simulink model "AS_H_Balanced_Load_7Bus"  (R2021a)
settings: Solver=ode45  StartTime=0.0  StopTime=1  RelTol=1e-3  EnableMultiTasking=on
undefined symbols (not defined in the file): D1, Delta
libraries: simulink_extras x12, spsDCVoltageSourceLib x12, spsDiodeLib x12, spsSeriesRLCBranchLib x12, spsGroundLib x10, spsRMSLib x8, dspstat3 x7, spsThreePhaseTransformerTwoWindingsLib x7, spsBreakerLib x7, spsThreePhaseSeriesRLCBranchLib x6, spsThreePhaseParallelRLCLoadLib x5, eePMU x4
(part 1 of 2)
settings Model: Creator=Gajanan-pc  LastModifiedBy=Hewlett-packard
settings SolverCC: AlgebraicLoopSolver=TrustRegion
settings DataIOCC: LimitDataPoints=on  SaveFormat=Array  ReturnWorkspaceOutputs=off
settings OptimizationCC: LifeSpan=inf
settings DebuggingCC: MaxConsecutiveZCsMsg=none  SolverPrmCheckMsg=warning  ParameterPrecisionLossMsg=none  SFUnexpectedBacktrackingDiag=warning  SFNoUnconditionalDefaultTransitionDiag=warning  SFExecutionAtInitializationDiag=none  SFMachineParentedDataDiag=warning  ArithmeticOperatorsInVariantConditions=warning
settings HardwareCC: ProdBitPerPointer=32  ProdBitPerSizeT=32  ProdBitPerPtrDiffT=32  ProdLargestAtomicFloat=None  ProdIntDivRoundTo=Undefined  ProdEndianess=Unspecified  ProdWordSize=32  ProdHWDeviceType=32-bit Generic
settings ModelReferenceCC: PropagateSignalLabelsOutOfModel=off
settings SFSimCC: SimUseLocalCustomCode=off  CustomCodeUndefinedFunction=UseInterfaceOnly
settings RTWCC: RTWUseLocalCustomCode=off
settings CodeAppCC: StateflowObjectComments=on
settings GRTTargetCC: TargetLangStandard=C89/C90 (ANSI)
settings ConfigComp: CovMetricSettings=dw  CovSaveCumulativeToWorkspaceVar=on  CovSaveSingleToWorkspaceVar=on  CovExternalEMLEnable=off  CovSFcnEnable=off
settings SimscapeCC: SimscapeNormalizeSystem=off

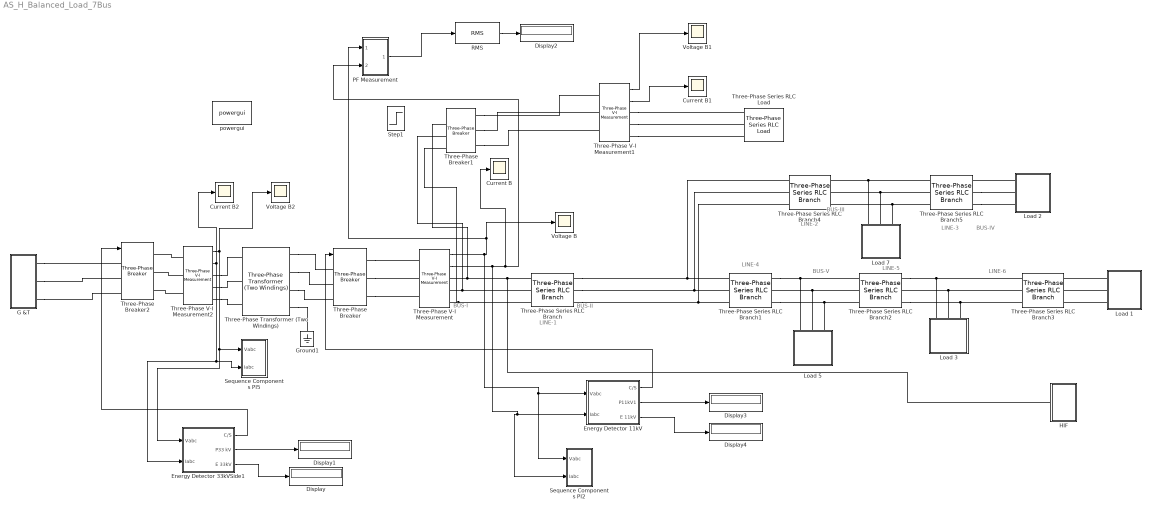
== system AS_H_Balanced_Load_7Bus ==
  note: LINE-1
  note: BUS-I
  note: BUS-II
  note: BUS-III
  note: BUS-IV
  note: BUS-V
  note: LINE-2
  note: LINE-3
  note: LINE-4
  note: LINE-5
  note: LINE-6
  Current B : Scope
  Current B1 : Scope
  Current B2 : Scope
  Display{,1..4} (5 alike) : Display
  Energy Detector 11kV : Subsystem
  Energy Detector 33kVSide1 : Subsystem
  G &T : Subsystem
  Ground1 : spsGroundLib/Ground  LConnTagsString=a
  HIF : Subsystem
  Load 1 : Subsystem
  Load 2 : Subsystem
  Load 3 : Subsystem
  Load 5 : Subsystem
  Load 7 : Subsystem
  PF Measurement : Subsystem
  RMS : dspstat3/RMS  run=off  directionMode=Each column  dimension=1  InputProcessing=Columns as channels (frame based)  reset_popup=None
  Sequence Components PI2 : Subsystem
  Sequence Components PI5 : Subsystem
  Step1 : Step  Time=0.8  SampleTime=0.1  ZeroCross=off
  Three-Phase Series RLC Branch : spsThreePhaseSeriesRLCBranchLib/Three-Phase Series RLC Branch  LConnTagsString=A|B|C  RConnTagsString=A|B|C  BranchType=RL  Resistance=0.2232  Inductance=0.012  Capacitance=0  Measurements=None
  Three-Phase Series RLC Branch1 : spsThreePhaseSeriesRLCBranchLib/Three-Phase Series RLC Branch  LConnTagsString=A|B|C  RConnTagsString=A|B|C  BranchType=RL  Resistance=0.9207  Inductance=0.0495  Capacitance=0  Measurements=None
  Three-Phase Series RLC Branch2 : spsThreePhaseSeriesRLCBranchLib/Three-Phase Series RLC Branch  LConnTagsString=A|B|C  RConnTagsString=A|B|C  BranchType=RL  Resistance=0.6138  Inductance=0.033  Capacitance=0  Measurements=None
  Three-Phase Series RLC Branch3 : spsThreePhaseSeriesRLCBranchLib/Three-Phase Series RLC Branch  LConnTagsString=A|B|C  RConnTagsString=A|B|C  BranchType=RL  Resistance=1.602  Inductance=0.057  Capacitance=0  Measurements=None
  Three-Phase Series RLC Branch4 : spsThreePhaseSeriesRLCBranchLib/Three-Phase Series RLC Branch  LConnTagsString=A|B|C  RConnTagsString=A|B|C  BranchType=RL  Resistance=0.7812  Inductance=0.042  Capacitance=0  Measurements=None
  Three-Phase Series RLC Branch5 : spsThreePhaseSeriesRLCBranchLib/Three-Phase Series RLC Branch  LConnTagsString=A|B|C  RConnTagsString=A|B|C  BranchType=RL  Resistance=1.1997  Inductance=0.0645  Capacitance=0  Measurements=None
  Three-Phase Series RLC Load : spsThreePhaseSeriesRLCLoadLib/Three-Phase Series RLC Load  LConnTagsString=A|B|C  Configuration=Y (floating)  NominalVoltage=12.65e3  Vabc=[1e3 1e3 1e3]  Vabcp=[1e3 1e3 1e3]  NominalFrequency=50  UnbalancedPower=off  ActivePower=0  InductivePower=108e3  CapacitivePower=1800e3  Pabc=[10e3 9e3 11e3]  QLabc=[100 90 110]  QCabc=[100 90 110]  Pabcp=[10e3 9e3 11e3]  QLabcp=[100 90 110]  QCabcp=[100 90 110]  Measurements=Branch voltages and currents  LoadType=constant PQ
  Three-Phase Transformer (Two Windings) : spsThreePhaseTransformerTwoWindingsLib/Three-Phase Transformer (Two Windings)  Winding1Connection=Delta (D1)  Winding2Connection=Yn  CoreType=Three-limb core (core-type)  SetSaturation=off  Hysteresis=off  DataFile='hysteresis'  SetInitialFlux=off  Measurements=None  UNITS=pu  NominalPower=[ 10e6 , 50 ]  Winding1=[33e3 , 0.002 , 0.08 ]  Winding2=[11e3 , 0.002 , 0.08 ]  Rm=500  Lm=500  L0=0.5  Saturation=[ 0,0 ; 0.0024,1.2 ; 1.0,1.52 ]  InitialFluxes=[-0.84855560977397 0.870082768362299 -0.0215271585931069]  BreakLoop=off  DiscreteSolver=Trapezoidal iterative  DataType=off  TransfoNumber=1
  Three-Phase V-I Measurement : spsThreePhaseVIMeasurementLib/Three-Phase V-I Measurement  VoltageMeasurement=phase-to-phase  SetLabelV=off  LabelV=Vabc  Vpu=off  VpuLL=off  CurrentMeasurement=yes  SetLabelI=off  LabelI=Iabc  Ipu=off  Pbase=100e6  Vbase=11e3  OutputType=Complex  PhasorSimulation=off  PSBequivalent=0
  Three-Phase V-I Measurement1 : spsThreePhaseVIMeasurementLib/Three-Phase V-I Measurement  VoltageMeasurement=phase-to-phase  SetLabelV=off  LabelV=Vabc  Vpu=off  VpuLL=off  CurrentMeasurement=yes  SetLabelI=off  LabelI=Iabc  Ipu=off  Pbase=100e6  Vbase=11e3  OutputType=Complex  PhasorSimulation=off  PSBequivalent=0
  Three-Phase V-I Measurement2 : spsThreePhaseVIMeasurementLib/Three-Phase V-I Measurement  VoltageMeasurement=phase-to-phase  SetLabelV=off  LabelV=Vabc  Vpu=off  VpuLL=off  CurrentMeasurement=yes  SetLabelI=off  LabelI=Iabc  Ipu=off  Pbase=100e6  Vbase=11e3  OutputType=Complex  PhasorSimulation=off  PSBequivalent=0
  Three-Phase Breaker : spsThreePhaseBreakerLib/Three-Phase Breaker  InitialState=closed  SwitchA=on  SwitchB=on  SwitchC=on  SwitchTimes=[1/50 5/50]  External=on  BreakerResistance=0.01  SnubberResistance=1e6  SnubberCapacitance=inf  Measurements=Breaker voltages and currents
  Three-Phase Breaker1 : spsThreePhaseBreakerLib/Three-Phase Breaker  InitialState=closed  SwitchA=on  SwitchB=on  SwitchC=on  SwitchTimes=[1/50 5/50]  External=on  BreakerResistance=0.01  SnubberResistance=1e6  SnubberCapacitance=inf  Measurements=Breaker voltages and currents
  Three-Phase Breaker2 : spsThreePhaseBreakerLib/Three-Phase Breaker  InitialState=closed  SwitchA=on  SwitchB=on  SwitchC=on  SwitchTimes=[1/50 5/50]  External=on  BreakerResistance=0.01  SnubberResistance=1e6  SnubberCapacitance=inf  Measurements=Breaker voltages and currents
  Voltage B : Scope
  Voltage B1 : Scope
  Voltage B2 : Scope
  powergui : spspowerguiLib/powergui  Priority=1  SimulationMode=Discrete  SampleTime=50e-6  frequency=60  Iterations=50  frequencyindice=0  Pbase=100e6  ErrMax=0.0001  UnitsV=kV  UnitsW=MW  buscounter=0  FunctionMessages=off  echomessages=off  EnableUseOfTLC=off  CurrentSourceSwitches=off  DisableSnubberDevices=off  DisableRonSwitches=off  DisableVfSwitches=off  DisplayEquations=off  AutomaticDiscreteSolvers=off  SolverType=Backward Euler  Interpol=off  ExternalGateDelay=off  methode=off  Ts=0  x0status=blocks  SPID=off  SwTol=0  HookPort=off  NonlinearTolerance=0  nMaxIteration=15  ContinueOnMaxIteration=off  RestoreLinks=warning  ResistiveCurrentMeasurement=off  Frange=[0:2:500]  Ylog=off  Xlog=on  ShowGrid=off  save=off  variable=ZData  structure=0  ZoomFFT=off  StartTime=0.0  cycles=1  DisplayStyle=1  fundamental=60  FreqAxis=off  MaxFrequency=1000  frequencyindicesteady=1  RmsSteady=1  display=off
  wires:
  Three-Phase V-I Measurement/2 -> Sequence Components PI2/2(Iabc), Energy Detector 11kV/2(Iabc), Current B/1, PF Measurement/2(In2)
  Three-Phase V-I Measurement1/1 -> Voltage B1/1
  Three-Phase V-I Measurement1/2 -> Current B1/1
  RMS/1 -> Display2/1
  PF Measurement/1(Out1) -> RMS/1
  Energy Detector 11kV/1(C/S) -> Three-Phase Breaker/1
  Three-Phase V-I Measurement/1 -> Sequence Components PI2/1(Vabc), Energy Detector 11kV/1(Vabc), Voltage B/1, PF Measurement/1(In1)
  Three-Phase V-I Measurement2/1 -> Sequence Components PI5/1(Vabc), Energy Detector 33kVSide1/1(Vabc), Voltage B2/1
  Three-Phase V-I Measurement2/2 -> Energy Detector 33kVSide1/2(Iabc), Sequence Components PI5/2(Iabc), Current B2/1
  Energy Detector 33kVSide1/1(C/S) -> Three-Phase Breaker2/1
  Energy Detector 33kVSide1/3(E 33kV) -> Display/1
  Energy Detector 33kVSide1/2(P33 kV) -> Display1/1
  Energy Detector 11kV/2(P11kV1) -> Display3/1
  Energy Detector 11kV/3(E 11kV) -> Display4/1
  connections:
  Three-Phase Series RLC Branch3/LConn2 -- Three-Phase Series RLC Branch2/RConn2 -- Load 3/LConn2
  Three-Phase Series RLC Branch2/RConn3 -- Load 3/LConn3 -- Three-Phase Series RLC Branch3/LConn3
  Three-Phase Series RLC Branch/LConn2 -- Three-Phase Breaker1/LConn2 -- Three-Phase V-I Measurement/RConn2
  Three-Phase Breaker/RConn2 -- Three-Phase V-I Measurement/LConn2
  Three-Phase Series RLC Branch/RConn3 -- Three-Phase Series RLC Branch1/LConn3 -- Three-Phase Series RLC Branch4/LConn3
  Three-Phase Series RLC Branch/LConn3 -- Three-Phase Breaker1/LConn3 -- Three-Phase V-I Measurement/RConn3
  Three-Phase Breaker/RConn1 -- Three-Phase V-I Measurement/LConn1
  Three-Phase Breaker/RConn3 -- Three-Phase V-I Measurement/LConn3
  Three-Phase Series RLC Branch5/LConn2 -- Load 7/LConn2 -- Three-Phase Series RLC Branch4/RConn2
  Three-Phase Series RLC Branch5/LConn3 -- Load 7/LConn3 -- Three-Phase Series RLC Branch4/RConn3
  Three-Phase Series RLC Branch/LConn1 -- HIF/LConn1 -- Three-Phase Breaker1/LConn1 -- Three-Phase V-I Measurement/RConn1
  Three-Phase Series RLC Branch1/RConn3 -- Three-Phase Series RLC Branch2/LConn3 -- Load 5/LConn3
  Three-Phase Series RLC Branch/RConn1 -- Three-Phase Series RLC Branch1/LConn1 -- Three-Phase Series RLC Branch4/LConn1
  Three-Phase V-I Measurement1/RConn1 -- Three-Phase Series RLC Load/LConn1
  Three-Phase V-I Measurement1/RConn2 -- Three-Phase Series RLC Load/LConn2
  Three-Phase V-I Measurement1/RConn3 -- Three-Phase Series RLC Load/LConn3
  Three-Phase Breaker1/RConn1 -- Three-Phase V-I Measurement1/LConn1
  Three-Phase Breaker1/RConn2 -- Three-Phase V-I Measurement1/LConn2
  Three-Phase Breaker1/RConn3 -- Three-Phase V-I Measurement1/LConn3
  Three-Phase Series RLC Branch2/LConn2 -- Load 5/LConn2 -- Three-Phase Series RLC Branch1/RConn2
  Three-Phase Series RLC Branch1/LConn2 -- Three-Phase Series RLC Branch4/LConn2 -- Three-Phase Series RLC Branch/RConn2
  Three-Phase Transformer (Two Windings)/RConn2 -- Three-Phase Breaker/LConn2
  Three-Phase Transformer (Two Windings)/RConn1 -- Three-Phase Breaker/LConn1
  Three-Phase Transformer (Two Windings)/RConn3 -- Three-Phase Breaker/LConn3
  Three-Phase Series RLC Branch5/LConn1 -- Three-Phase Series RLC Branch4/RConn1 -- Load 7/LConn1
  Load 1/LConn2 -- Three-Phase Series RLC Branch3/RConn2
  Load 1/LConn3 -- Three-Phase Series RLC Branch3/RConn3
  Load 2/LConn1 -- Three-Phase Series RLC Branch5/RConn1
  Three-Phase Series RLC Branch5/RConn2 -- Load 2/LConn2
  Three-Phase Series RLC Branch5/RConn3 -- Load 2/LConn3
  Three-Phase Transformer (Two Windings)/RConn4 -- Ground1/LConn1
  Load 1/LConn1 -- Three-Phase Series RLC Branch3/RConn1
  Load 5/LConn1 -- Three-Phase Series RLC Branch1/RConn1 -- Three-Phase Series RLC Branch2/LConn1
  Three-Phase V-I Measurement2/LConn1 -- Three-Phase Breaker2/RConn1
  Three-Phase V-I Measurement2/LConn2 -- Three-Phase Breaker2/RConn2
  Three-Phase V-I Measurement2/LConn3 -- Three-Phase Breaker2/RConn3
  Three-Phase V-I Measurement2/RConn1 -- Three-Phase Transformer (Two Windings)/LConn1
  Three-Phase V-I Measurement2/RConn2 -- Three-Phase Transformer (Two Windings)/LConn2
  Three-Phase V-I Measurement2/RConn3 -- Three-Phase Transformer (Two Windings)/LConn3
  G &T/RConn1 -- Three-Phase Breaker2/LConn1
  G &T/RConn2 -- Three-Phase Breaker2/LConn2
  G &T/RConn3 -- Three-Phase Breaker2/LConn3
  Three-Phase Series RLC Branch2/RConn1 -- Load 3/LConn1 -- Three-Phase Series RLC Branch3/LConn1

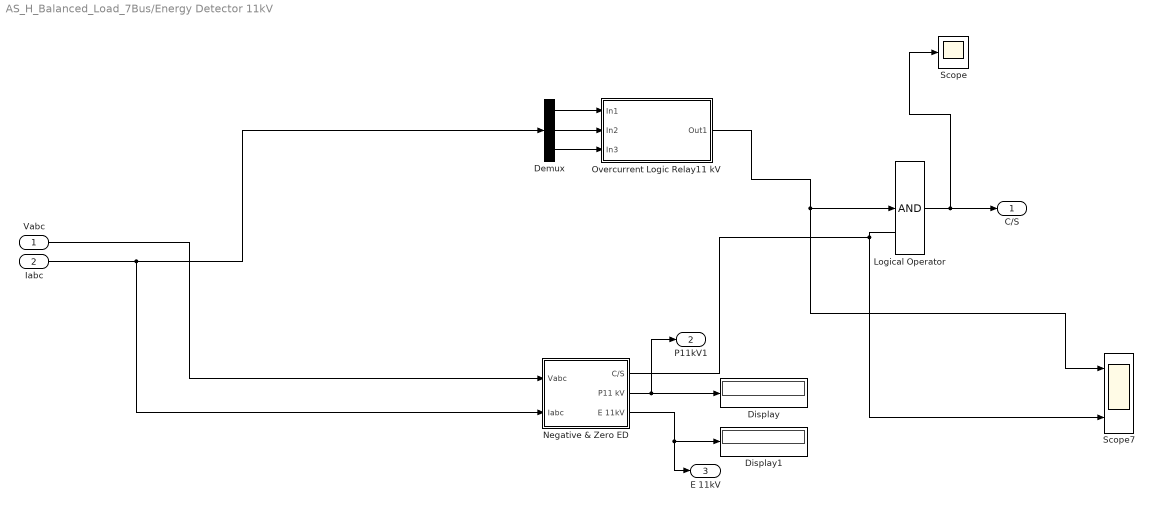
== system AS_H_Balanced_Load_7Bus/Energy Detector 11kV ==
  Vabc : Inport
  Iabc : Inport  Port=2
  Demux : Demux  Outputs=3
  Display : Display
  Display1 : Display
  Logical Operator : Logic  Inputs=1  AllPortsSameDT=off
  "Negative & Zero ED " : Subsystem
  "Overcurrent Logic Relay11 kV " : Subsystem  TreatAsAtomicUnit=on
  Scope : Scope
  Scope7 : Scope  NumInputPorts=3
  C/S : Outport  VectorParamsAs1DForOutWhenUnconnected=off
  P11kV1 : Outport  Port=2  VectorParamsAs1DForOutWhenUnconnected=off
  E 11kV : Outport  Port=3  VectorParamsAs1DForOutWhenUnconnected=off
  wires:
  Iabc/1 -> "Negative & Zero ED "/2(Iabc), Demux/1
  Demux/3 -> "Overcurrent Logic Relay11 kV "/3(In3)
  Demux/1 -> "Overcurrent Logic Relay11 kV "/1(In1)
  Demux/2 -> "Overcurrent Logic Relay11 kV "/2(In2)
  "Overcurrent Logic Relay11 kV "/1(Out1) -> Scope7/1, Logical Operator/1
  Logical Operator/1 -> Scope/1, C/S/1
  Vabc/1 -> "Negative & Zero ED "/1(Vabc)
  "Negative & Zero ED "/1(C/S) -> Scope7/3
  "Negative & Zero ED "/2(P11 kV) -> Display/1, P11kV1/1
  "Negative & Zero ED "/3(E 11kV) -> E 11kV/1, Display1/1

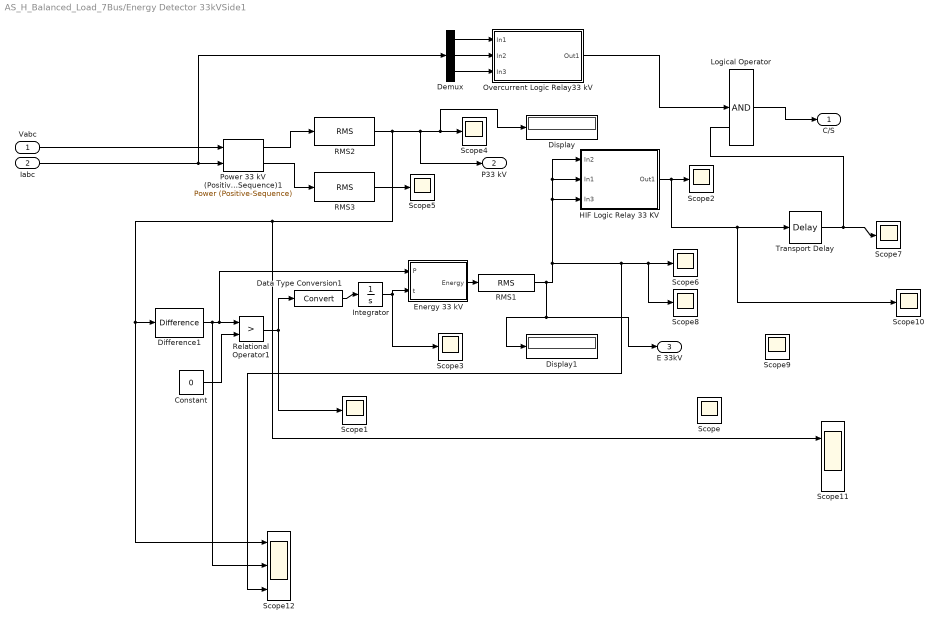
== system AS_H_Balanced_Load_7Bus/Energy Detector 33kVSide1 ==
  Vabc : Inport
  Iabc : Inport  Port=2
  Constant : Constant  Value=0
  Data Type Conversion1 : DataTypeConversion
  Demux : Demux  Outputs=3
  Difference1 : simulink/Discrete/Difference  ICPrevInput=0.0  OutMin=[]  OutMax=[]  OutDataType=fixdt(1, 16)  OutScaling=2^-10  DoSatur=off
  Display : Display
  Display1 : Display
  Energy 33 kV : MATLAB Function  TreatAsAtomicUnit=on
  HIF Logic Relay 33 KV : Subsystem  TreatAsAtomicUnit=on
  Integrator : Integrator
  Logical Operator : Logic  Inputs=1  AllPortsSameDT=off
  Overcurrent Logic Relay33 kV : Subsystem  TreatAsAtomicUnit=on
  Power 33 kV (Positive-Sequence)1 : spsPowerPositiveSequenceLib/Power (Positive-Sequence)  Freq=50  Vinit=[0, 0]  Iinit=[0, 0]  Ts=0
      link override Sequence Analyzer: Freq=50  seq=Negative
      link override Sequence Analyzer1: Freq=50  seq=Negative
      settings: SourceProductBaseCode=PS
  RMS1 : dspstat3/RMS  run=off  directionMode=Each column  dimension=1  InputProcessing=Columns as channels (frame based)  reset_popup=None
  RMS2 : dspstat3/RMS  run=off  directionMode=Each column  dimension=1  InputProcessing=Columns as channels (frame based)  reset_popup=None
  RMS3 : dspstat3/RMS  run=off  directionMode=Each column  dimension=1  InputProcessing=Columns as channels (frame based)  reset_popup=None
  Relational Operator1 : RelationalOperator  Operator=>  RndMeth=Nearest
  Scope{,1..10} (11 alike) : Scope
  Scope11 : Scope  NumInputPorts=2
  Scope12 : Scope  NumInputPorts=3
  Transport Delay : TransportDelay  DelayTime=0.1  InitialOutput=1
  C/S : Outport  VectorParamsAs1DForOutWhenUnconnected=off
  P33 kV : Outport  Port=2  VectorParamsAs1DForOutWhenUnconnected=off
  E 33kV : Outport  Port=3  VectorParamsAs1DForOutWhenUnconnected=off
  wires:
  Power 33 kV (Positive-Sequence)1/2 -> RMS3/1
  Iabc/1 -> Demux/1, Power 33 kV (Positive-Sequence)1/2
  Demux/3 -> Overcurrent Logic Relay33 kV/3(In3)
  RMS3/1 -> Scope5/1
  Demux/1 -> Overcurrent Logic Relay33 kV/1(In1)
  Energy 33 kV/1(Energy) -> RMS1/1
  Integrator/1 -> Scope3/1, Energy 33 kV/2(t)
  Power 33 kV (Positive-Sequence)1/1 -> RMS2/1
  Demux/2 -> Overcurrent Logic Relay33 kV/2(In2)
  Overcurrent Logic Relay33 kV/1(Out1) -> Logical Operator/1
  Vabc/1 -> Power 33 kV (Positive-Sequence)1/1
  Logical Operator/1 -> C/S/1
  Data Type Conversion1/1 -> Integrator/1
  Relational Operator1/1 -> Data Type Conversion1/1, Scope1/1
  RMS2/1 -> Scope11/1, Scope12/1, Difference1/1, P33 kV/1, Scope4/1, Display/1
  HIF Logic Relay 33 KV/1(Out1) -> Scope10/1, Transport Delay/1, Scope2/1
  Transport Delay/1 -> Scope7/1
  Constant/1 -> Relational Operator1/2
  Difference1/1 -> Scope12/2, Energy 33 kV/1(P), Relational Operator1/1
  RMS1/1 -> Display1/1, E 33kV/1, Scope12/3, Scope8/1, Scope6/1, HIF Logic Relay 33 KV/3(In3), HIF Logic Relay 33 KV/2(In1), HIF Logic Relay 33 KV/1(In2)

== system AS_H_Balanced_Load_7Bus/G &T ==
  Ground2 : spsGroundLib/Ground  LConnTagsString=a
  Ground3 : spsGroundLib/Ground  LConnTagsString=a
  Ground4 : spsGroundLib/Ground  LConnTagsString=a
  Three-Phase Programmable Voltage Source1 : spsThreePhaseProgrammableVoltageSourceLib/Three-Phase Programmable Voltage Source  PositiveSequence="[220e3  0 50]"  VariationEntity=None  VariationType=Table of time-amplitude pairs  VariationTypeAlt=Step  VariationStep=0.5  VariationRate=10  VariationMagnitude=0.3  VariationFrequency=2  VariationTiming=[.01 .05 1]  VariationPhaseA=off  Amplitudes=[1 0.8 1.2 1.0]  TimeValues=[0 0.1 0.15 0.2]  HarmonicGeneration=off  HarmonicA=[3 0.2 -25 0]  HarmonicB=[2 0.15 35 2]  Timing="[0.05  3]"  BusType=PQ  Pref=5e6  Qref=0  Qmin=0.5e6  Qmax=0
  Three-Phase Transformer (Two Windings)1 : spsThreePhaseTransformerTwoWindingsLib/Three-Phase Transformer (Two Windings)  Winding1Connection=Yn  Winding2Connection=Yn  CoreType=Three-limb core (core-type)  SetSaturation=off  Hysteresis=off  DataFile='hysteresis'  SetInitialFlux=off  Measurements=All measurements (V I Fluxes)  UNITS=pu  NominalPower=[ 50e6 , 50 ]  Winding1=[2.2e+05 0.002 0.08]  Winding2=[33000 0.002 0.08]  Rm=500  Lm=499.99  L0=0.49999  Saturation=[0 0;0.0024 1.2;1 1.52]  InitialFluxes=[-0.991141122701691 0.498581403361155 0.49255971934211]  BreakLoop=off  DiscreteSolver=Trapezoidal iterative  DataType=off  TransfoNumber=1
  a : PMIOPort  Side=Right
  b : PMIOPort  Port=2  Side=Right
  c : PMIOPort  Port=3  Side=Right
  connections:
  Ground3/LConn1 -- Three-Phase Programmable Voltage Source1/LConn1
  Three-Phase Transformer (Two Windings)1/RConn1 -- a/RConn1
  Ground2/LConn1 -- Three-Phase Transformer (Two Windings)1/LConn4
  Three-Phase Programmable Voltage Source1/RConn3 -- Three-Phase Transformer (Two Windings)1/LConn3
  Three-Phase Programmable Voltage Source1/RConn2 -- Three-Phase Transformer (Two Windings)1/LConn2
  Three-Phase Programmable Voltage Source1/RConn1 -- Three-Phase Transformer (Two Windings)1/LConn1
  Ground4/LConn1 -- Three-Phase Transformer (Two Windings)1/RConn4
  Three-Phase Transformer (Two Windings)1/RConn2 -- b/RConn1
  Three-Phase Transformer (Two Windings)1/RConn3 -- c/RConn1

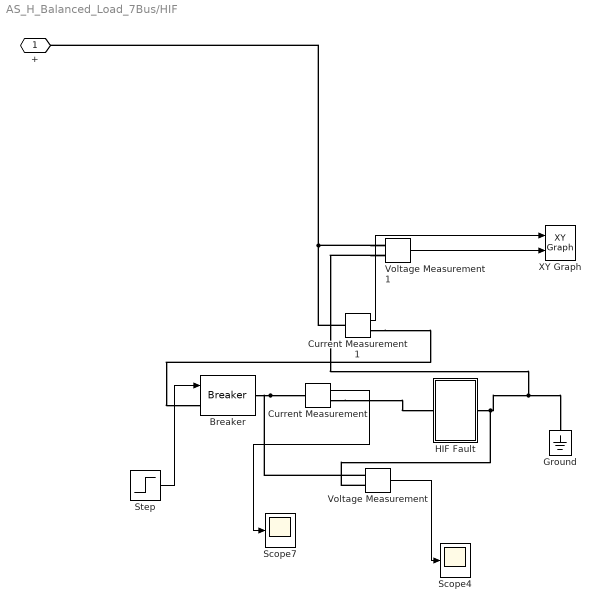
== system AS_H_Balanced_Load_7Bus/HIF ==
  Breaker : spsBreakerLib/Breaker  InitialState=0  SwitchingTimes="[1/50  5/50]"  External=on  BreakerResistance=0.01  SnubberResistance=1e6  SnubberCapacitance=inf  Measurements=Branch voltage and current  MoreParameters=on  NoBreakLoop=off
      settings: SourceProductBaseCode=PS
  Current Measurement : spsCurrentMeasurementLib/Current Measurement  PhasorSimulation=off  OutputType=Complex  PSBequivalent=0
  Current Measurement1 : spsCurrentMeasurementLib/Current Measurement  PhasorSimulation=off  OutputType=Complex  PSBequivalent=0
  Ground : spsGroundLib/Ground  LConnTagsString=a
  HIF Fault : Subsystem
  Scope4 : Scope
  Scope7 : Scope
  Step : Step  Time=0.9  SampleTime=0.1  ZeroCross=off
  Voltage Measurement : spsVoltageMeasurementLib/Voltage Measurement  PhasorSimulation=off  OutputType=Complex  PSBequivalent=0
  Voltage Measurement1 : spsVoltageMeasurementLib/Voltage Measurement  PhasorSimulation=off  OutputType=Complex  PSBequivalent=0
  XY Graph : simulink/Sinks/XY Graph  xmin=-100  xmax=100  ymin=-7000  ymax=7000  st=-1
  + : PMIOPort  Side=Left
  wires:
  Current Measurement/1 -> Scope7/1
  Step/1 -> Breaker/1
  Voltage Measurement/1 -> Scope4/1
  Current Measurement1/1 -> XY Graph/1
  Voltage Measurement1/1 -> XY Graph/2
  connections:
  Current Measurement1/LConn1 -- +/RConn1 -- Voltage Measurement1/LConn1
  HIF Fault/RConn1 -- Voltage Measurement/LConn2 -- Voltage Measurement1/LConn2 -- Ground/LConn1
  Voltage Measurement/LConn1 -- Breaker/RConn1 -- Current Measurement/LConn1
  Current Measurement/RConn1 -- HIF Fault/LConn1
  Current Measurement1/RConn1 -- Breaker/LConn1

== system AS_H_Balanced_Load_7Bus/Load 1 ==
  Ground : spsGroundLib/Ground  LConnTagsString=a
  Three-Phase Parallel RLC Load2 : spsThreePhaseParallelRLCLoadLib/Three-Phase Parallel RLC Load  LConnTagsString=A|B|C  RConnTagsString=N  Configuration=Y (neutral)  NominalVoltage=[248 248 248]  Vabc=[248 248 248]  Vabcp=[1e3 1e3 1e3]  NominalFrequency=50  UnbalancedPower=on  ActivePower=10e3  InductivePower=100  CapacitivePower=100  Pabc=[645e3 645e3 645e3]  QLabc=[312e3 312e3 312e3]  QCabc=[0 0 0]  Pabcp=[10e3 9e3 11e3]  QLabcp=[100 90 110]  QCabcp=[100 90 110]  Measurements=Branch voltages and currents  LoadType=constant Z
  Three-Phase Transformer (Two Windings)2 : spsThreePhaseTransformerTwoWindingsLib/Three-Phase Transformer (Two Windings)  Winding1Connection=Delta (D1)  Winding2Connection=Yn  CoreType=Three-limb core (core-type)  SetSaturation=off  Hysteresis=off  DataFile='hysteresis'  SetInitialFlux=off  Measurements=All measurements (V I Fluxes)  UNITS=pu  NominalPower=[ 0.5e6 , 50 ]  Winding1=[11e3 , 0.002 , 0.08 ]  Winding2=[433 , 0.002 , 0.08 ]  Rm=250  Lm=250  L0=0.5  Saturation=[ 0,0 ; 0.0024,1.2 ; 1.0,1.52 ]  InitialFluxes=[0.167363107089062 0.0610185437238888 -0.245329692895651]  BreakLoop=off  DiscreteSolver=Trapezoidal iterative  DataType=off  TransfoNumber=1
  A : PMIOPort  Side=Left
  B : PMIOPort  Port=2  Side=Left
  C : PMIOPort  Port=3  Side=Left
  connections:
  Three-Phase Transformer (Two Windings)2/LConn2 -- B/RConn1
  Three-Phase Transformer (Two Windings)2/LConn3 -- C/RConn1
  Three-Phase Transformer (Two Windings)2/LConn1 -- A/RConn1
  Three-Phase Parallel RLC Load2/LConn1 -- Three-Phase Transformer (Two Windings)2/RConn1
  Three-Phase Parallel RLC Load2/LConn2 -- Three-Phase Transformer (Two Windings)2/RConn2
  Three-Phase Parallel RLC Load2/LConn3 -- Three-Phase Transformer (Two Windings)2/RConn3
  Three-Phase Parallel RLC Load2/RConn1 -- Three-Phase Transformer (Two Windings)2/RConn4 -- Ground/LConn1

== system AS_H_Balanced_Load_7Bus/Load 2 ==
  Ground : spsGroundLib/Ground  LConnTagsString=a
  Three-Phase Parallel RLC Load2 : spsThreePhaseParallelRLCLoadLib/Three-Phase Parallel RLC Load  LConnTagsString=A|B|C  RConnTagsString=N  Configuration=Y (neutral)  NominalVoltage=[248 248 248]  Vabc=[248 248 248]  Vabcp=[1e3 1e3 1e3]  NominalFrequency=50  UnbalancedPower=on  ActivePower=10e3  InductivePower=100  CapacitivePower=100  Pabc=[145e3 145e3 145e3]  QLabc=[28e3 28e3 28e3]  QCabc=[0 0 0]  Pabcp=[10e3 9e3 11e3]  QLabcp=[100 90 110]  QCabcp=[100 90 110]  Measurements=Branch voltages and currents  LoadType=constant Z
  Three-Phase Transformer (Two Windings)2 : spsThreePhaseTransformerTwoWindingsLib/Three-Phase Transformer (Two Windings)  Winding1Connection=Delta (D1)  Winding2Connection=Yn  CoreType=Three-limb core (core-type)  SetSaturation=off  Hysteresis=off  DataFile='hysteresis'  SetInitialFlux=off  Measurements=All measurements (V I Fluxes)  UNITS=pu  NominalPower=[1e3 , 50 ]  Winding1=[11e3 , 0.002 , 0.08 ]  Winding2=[433 , 0.002 , 0.08 ]  Rm=250  Lm=250  L0=0.5  Saturation=[ 0,0 ; 0.0024,1.2 ; 1.0,1.52 ]  InitialFluxes=[-0.093644263507764 0.838815084304348 -0.653451497613207]  BreakLoop=off  DiscreteSolver=Trapezoidal iterative  DataType=off  TransfoNumber=1
  A : PMIOPort  Side=Left
  B : PMIOPort  Port=2  Side=Left
  C : PMIOPort  Port=3  Side=Left
  connections:
  Three-Phase Transformer (Two Windings)2/LConn2 -- B/RConn1
  Three-Phase Transformer (Two Windings)2/LConn3 -- C/RConn1
  Three-Phase Transformer (Two Windings)2/LConn1 -- A/RConn1
  Three-Phase Transformer (Two Windings)2/RConn4 -- Three-Phase Parallel RLC Load2/RConn1 -- Ground/LConn1
  Three-Phase Transformer (Two Windings)2/RConn1 -- Three-Phase Parallel RLC Load2/LConn1
  Three-Phase Transformer (Two Windings)2/RConn2 -- Three-Phase Parallel RLC Load2/LConn2
  Three-Phase Transformer (Two Windings)2/RConn3 -- Three-Phase Parallel RLC Load2/LConn3

== system AS_H_Balanced_Load_7Bus/Load 3 ==
  Ground : spsGroundLib/Ground  LConnTagsString=a
  Three-Phase Parallel RLC Load2 : spsThreePhaseParallelRLCLoadLib/Three-Phase Parallel RLC Load  LConnTagsString=A|B|C  RConnTagsString=N  Configuration=Y (neutral)  NominalVoltage=[248 248 248]  Vabc=[248 248 248]  Vabcp=[1e3 1e3 1e3]  NominalFrequency=50  UnbalancedPower=on  ActivePower=10e3  InductivePower=100  CapacitivePower=100  Pabc=[432e3 432e3 432e3]  QLabc=[103e3 103e3 103e3]  QCabc=[0 0 0]  Pabcp=[10e3 9e3 11e3]  QLabcp=[100 90 110]  QCabcp=[100 90 110]  Measurements=Branch voltages and currents  LoadType=constant Z
  Three-Phase Transformer (Two Windings)2 : spsThreePhaseTransformerTwoWindingsLib/Three-Phase Transformer (Two Windings)  Winding1Connection=Delta (D1)  Winding2Connection=Yn  CoreType=Three-limb core (core-type)  SetSaturation=off  Hysteresis=off  DataFile='hysteresis'  SetInitialFlux=off  Measurements=All measurements (V I Fluxes)  UNITS=pu  NominalPower=[ 0.5e6 , 50 ]  Winding1=[11e3 , 0.002 , 0.08 ]  Winding2=[ 433 , 0.002 , 0.08 ]  Rm=250  Lm=250  L0=0.5  Saturation=[ 0,0 ; 0.0024,1.2 ; 1.0,1.52 ]  InitialFluxes=[0.177589955789988 0.125733120517853 -0.299711964168377]  BreakLoop=off  DiscreteSolver=Trapezoidal iterative  DataType=off  TransfoNumber=1
  A : PMIOPort  Side=Left
  B : PMIOPort  Port=2  Side=Left
  C : PMIOPort  Port=3  Side=Left
  connections:
  Three-Phase Transformer (Two Windings)2/LConn2 -- B/RConn1
  Three-Phase Transformer (Two Windings)2/LConn3 -- C/RConn1
  Three-Phase Transformer (Two Windings)2/LConn1 -- A/RConn1
  Three-Phase Parallel RLC Load2/LConn1 -- Three-Phase Transformer (Two Windings)2/RConn1
  Three-Phase Transformer (Two Windings)2/RConn2 -- Three-Phase Parallel RLC Load2/LConn2
  Three-Phase Transformer (Two Windings)2/RConn3 -- Three-Phase Parallel RLC Load2/LConn3
  Three-Phase Transformer (Two Windings)2/RConn4 -- Three-Phase Parallel RLC Load2/RConn1 -- Ground/LConn1

== system AS_H_Balanced_Load_7Bus/Load 5 ==
  Ground : spsGroundLib/Ground  LConnTagsString=a
  Three-Phase Parallel RLC Load1 : spsThreePhaseParallelRLCLoadLib/Three-Phase Parallel RLC Load  LConnTagsString=A|B|C  RConnTagsString=N  Configuration=Y (neutral)  NominalVoltage=[248 248 248]  Vabc=[248 248 248]  Vabcp=[1e3 1e3 1e3]  NominalFrequency=50  UnbalancedPower=on  ActivePower=10e3  InductivePower=100  CapacitivePower=100  Pabc=[732e3 732e3 732e3]  QLabc=[112e3 112e3 112e3]  QCabc=[0 0 0]  Pabcp=[10e3 9e3 11e3]  QLabcp=[100 90 110]  QCabcp=[100 90 110]  Measurements=Branch voltages and currents  LoadType=constant Z
  Three-Phase Transformer (Two Windings)2 : spsThreePhaseTransformerTwoWindingsLib/Three-Phase Transformer (Two Windings)  Winding1Connection=Delta (D1)  Winding2Connection=Yn  CoreType=Three-limb core (core-type)  SetSaturation=off  Hysteresis=off  DataFile='hysteresis'  SetInitialFlux=off  Measurements=All measurements (V I Fluxes)  UNITS=pu  NominalPower=[ 1e6 , 50 ]  Winding1=[ 11e3 , 0.002 , 0.08 ]  Winding2=[ 433 , 0.002 , 0.08 ]  Rm=250  Lm=250  L0=0.5  Saturation=[ 0,0 ; 0.0024,1.2 ; 1.0,1.52 ]  InitialFluxes=[-0.0247540799705537 0.677855009969254 -0.599270009227358]  BreakLoop=off  DiscreteSolver=Trapezoidal iterative  DataType=off  TransfoNumber=1
  A : PMIOPort  Side=Left
  B : PMIOPort  Port=2  Side=Left
  C : PMIOPort  Port=3  Side=Left
  connections:
  Three-Phase Transformer (Two Windings)2/LConn1 -- A/RConn1
  Three-Phase Transformer (Two Windings)2/LConn3 -- C/RConn1
  Three-Phase Transformer (Two Windings)2/LConn2 -- B/RConn1
  Three-Phase Parallel RLC Load1/LConn1 -- Three-Phase Transformer (Two Windings)2/RConn1
  Three-Phase Transformer (Two Windings)2/RConn2 -- Three-Phase Parallel RLC Load1/LConn2
  Three-Phase Transformer (Two Windings)2/RConn3 -- Three-Phase Parallel RLC Load1/LConn3
  Three-Phase Transformer (Two Windings)2/RConn4 -- Three-Phase Parallel RLC Load1/RConn1 -- Ground/LConn1

== system AS_H_Balanced_Load_7Bus/Load 7 ==
  Ground : spsGroundLib/Ground  LConnTagsString=a
  Three-Phase Parallel RLC Load1 : spsThreePhaseParallelRLCLoadLib/Three-Phase Parallel RLC Load  LConnTagsString=A|B|C  RConnTagsString=N  Configuration=Y (neutral)  NominalVoltage=[248 248 248]  Vabc=[248 248 248]  Vabcp=[1e3 1e3 1e3]  NominalFrequency=50  UnbalancedPower=on  ActivePower=10e3  InductivePower=100  CapacitivePower=100  Pabc=[643e3 643e3 643e3]  QLabc=[100e3 100e3 100e3]  QCabc=[0 0 0]  Pabcp=[10e3 9e3 11e3]  QLabcp=[100 90 110]  QCabcp=[100 90 110]  Measurements=Branch voltages and currents  LoadType=constant Z
  Three-Phase Transformer (Two Windings)2 : spsThreePhaseTransformerTwoWindingsLib/Three-Phase Transformer (Two Windings)  Winding1Connection=Delta (D1)  Winding2Connection=Yn  CoreType=Three-limb core (core-type)  SetSaturation=off  Hysteresis=off  DataFile='hysteresis'  SetInitialFlux=off  Measurements=All measurements (V I Fluxes)  UNITS=SI  NominalPower=[1e6 , 50 ]  Winding1=[11e3 0.002 0.08]  Winding2=[433 0.002 0.08]  Rm=250  Lm=250  L0=0.36108  Saturation=[0 0;0.16456 59.421;68.568 75.266]  InitialFluxes=[-5.25282919688326 40.1491552037539 -34.8961082612815]  BreakLoop=off  DiscreteSolver=Trapezoidal iterative  DataType=on  TransfoNumber=1
  A : PMIOPort  Side=Left
  B : PMIOPort  Port=2  Side=Left
  C : PMIOPort  Port=3  Side=Left
  connections:
  Three-Phase Transformer (Two Windings)2/LConn2 -- B/RConn1
  Three-Phase Transformer (Two Windings)2/LConn3 -- C/RConn1
  Three-Phase Transformer (Two Windings)2/LConn1 -- A/RConn1
  Three-Phase Parallel RLC Load1/LConn1 -- Three-Phase Transformer (Two Windings)2/RConn1
  Three-Phase Transformer (Two Windings)2/RConn2 -- Three-Phase Parallel RLC Load1/LConn2
  Three-Phase Transformer (Two Windings)2/RConn3 -- Three-Phase Parallel RLC Load1/LConn3
  Three-Phase Transformer (Two Windings)2/RConn4 -- Three-Phase Parallel RLC Load1/RConn1 -- Ground/LConn1

== system AS_H_Balanced_Load_7Bus/PF Measurement ==
  In1 : Inport
  In2 : Inport  Port=2
  Divide : Product  Inputs=*/
  "Power (3ph, Instantaneous)" : spsPower3phInstantaneousLib/Power (3ph, Instantaneous)
  Product : Product
  Product2 : Product
  Square Root : Sqrt  SaturateOnIntegerOverflow=on
  Sum : Sum  Inputs=|++
  Out1 : Outport  VectorParamsAs1DForOutWhenUnconnected=off
  wires:
  "Power (3ph, Instantaneous)"/1 -> Divide/1, Product/2, Product/1
  In2/1 -> "Power (3ph, Instantaneous)"/2
  Product2/1 -> Sum/2
  Sum/1 -> Square Root/1
  In1/1 -> "Power (3ph, Instantaneous)"/1
  "Power (3ph, Instantaneous)"/2 -> Product2/2, Product2/1
  Product/1 -> Sum/1
  Square Root/1 -> Divide/2
  Divide/1 -> Out1/1

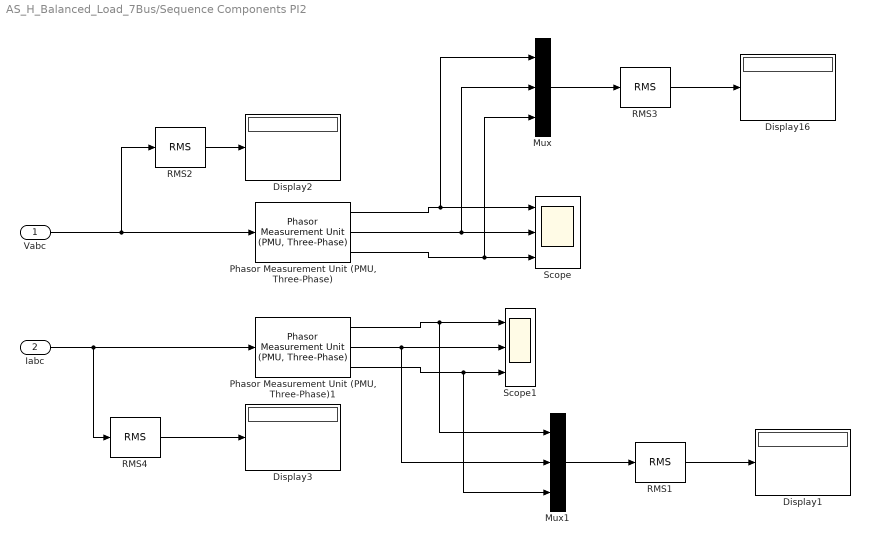
== system AS_H_Balanced_Load_7Bus/Sequence Components PI2 ==
  Vabc : Inport
  Iabc : Inport  Port=2
  Display{1..3,16} (4 alike) : Display
  Mux : Mux  Inputs=3
  Mux1 : Mux  Inputs=3
  "Phasor Measurement Unit (PMU, Three-Phase)" : eePMU/Phasor Measurement Unit (PMU, Three-Phase)  frequency=50  Nsr=64  k=1
      settings: SourceProductBaseCode=PS
  "Phasor Measurement Unit (PMU, Three-Phase)1" : eePMU/Phasor Measurement Unit (PMU, Three-Phase)  frequency=50  Nsr=64  k=1
      settings: SourceProductBaseCode=PS
  RMS{1..4} (4 alike) : spsRMSLib/RMS  TrueRMS=on  Freq=50  RMSInit=0  Ts=0
  Scope : Scope  NumInputPorts=3
  Scope1 : Scope  NumInputPorts=3
  wires:
  RMS3/1 -> Display16/1
  RMS1/1 -> Display1/1
  RMS2/1 -> Display2/1
  Vabc/1 -> "Phasor Measurement Unit (PMU, Three-Phase)"/1, RMS2/1
  RMS4/1 -> Display3/1
  Iabc/1 -> "Phasor Measurement Unit (PMU, Three-Phase)1"/1, RMS4/1
  "Phasor Measurement Unit (PMU, Three-Phase)"/1 -> Scope/1, Mux/1
  "Phasor Measurement Unit (PMU, Three-Phase)"/2 -> Scope/2, Mux/2
  "Phasor Measurement Unit (PMU, Three-Phase)"/3 -> Scope/3, Mux/3
  "Phasor Measurement Unit (PMU, Three-Phase)1"/1 -> Scope1/1, Mux1/1
  "Phasor Measurement Unit (PMU, Three-Phase)1"/2 -> Scope1/2, Mux1/2
  "Phasor Measurement Unit (PMU, Three-Phase)1"/3 -> Scope1/3, Mux1/3
  Mux/1 -> RMS3/1
  Mux1/1 -> RMS1/1

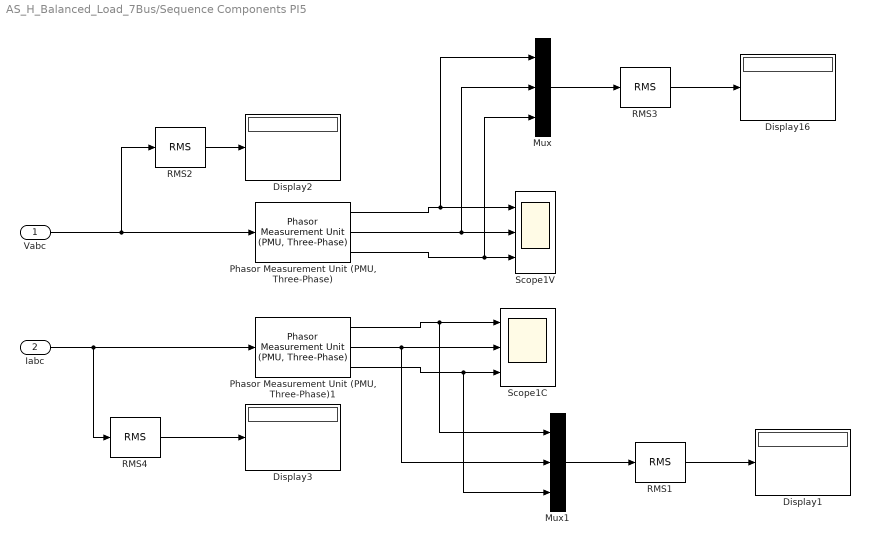
== system AS_H_Balanced_Load_7Bus/Sequence Components PI5 ==
  Vabc : Inport
  Iabc : Inport  Port=2
  Display{1..3,16} (4 alike) : Display
  Mux : Mux  Inputs=3
  Mux1 : Mux  Inputs=3
  "Phasor Measurement Unit (PMU, Three-Phase)" : eePMU/Phasor Measurement Unit (PMU, Three-Phase)  frequency=50  Nsr=64  k=1
      settings: SourceProductBaseCode=PS
  "Phasor Measurement Unit (PMU, Three-Phase)1" : eePMU/Phasor Measurement Unit (PMU, Three-Phase)  frequency=50  Nsr=64  k=1
      settings: SourceProductBaseCode=PS
  RMS{1..4} (4 alike) : spsRMSLib/RMS  TrueRMS=on  Freq=50  RMSInit=0  Ts=0
  Scope1C : Scope  NumInputPorts=3
  Scope1V : Scope  NumInputPorts=3
  wires:
  RMS3/1 -> Display16/1
  RMS1/1 -> Display1/1
  RMS2/1 -> Display2/1
  Vabc/1 -> "Phasor Measurement Unit (PMU, Three-Phase)"/1, RMS2/1
  RMS4/1 -> Display3/1
  Iabc/1 -> "Phasor Measurement Unit (PMU, Three-Phase)1"/1, RMS4/1
  "Phasor Measurement Unit (PMU, Three-Phase)"/1 -> Mux/1, Scope1V/1
  "Phasor Measurement Unit (PMU, Three-Phase)"/2 -> Mux/2, Scope1V/2
  "Phasor Measurement Unit (PMU, Three-Phase)"/3 -> Mux/3, Scope1V/3
  "Phasor Measurement Unit (PMU, Three-Phase)1"/1 -> Mux1/1, Scope1C/1
  "Phasor Measurement Unit (PMU, Three-Phase)1"/2 -> Mux1/2, Scope1C/2
  "Phasor Measurement Unit (PMU, Three-Phase)1"/3 -> Mux1/3, Scope1C/3
  Mux/1 -> RMS3/1
  Mux1/1 -> RMS1/1

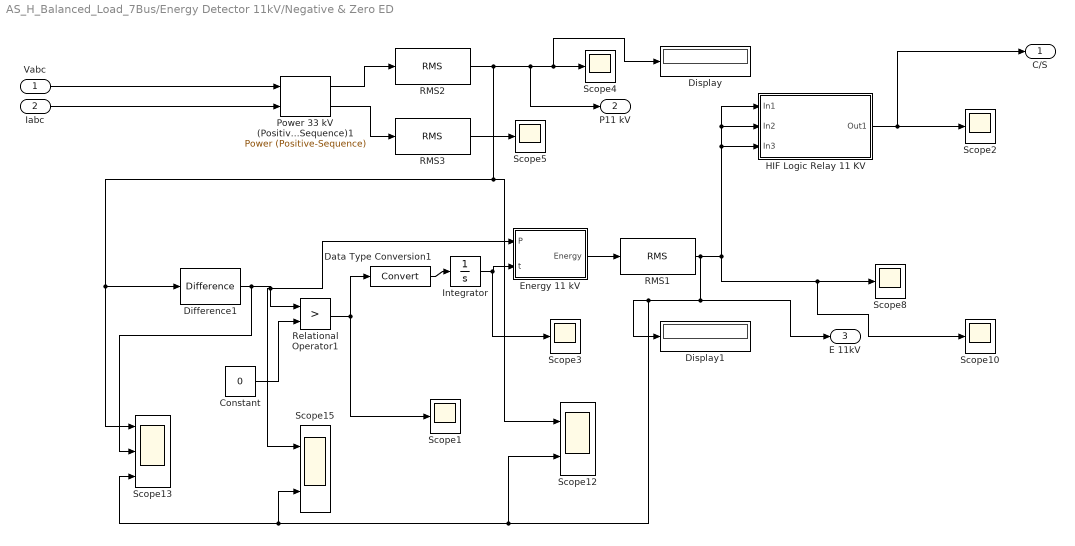
== system AS_H_Balanced_Load_7Bus/Energy Detector 11kV/Negative & Zero ED  ==
  Vabc : Inport
  Iabc : Inport  Port=2
  Constant : Constant  Value=0
  Data Type Conversion1 : DataTypeConversion
  Difference1 : simulink/Discrete/Difference  ICPrevInput=0.0  OutMin=[]  OutMax=[]  OutDataType=fixdt(1, 16)  OutScaling=2^-10  DoSatur=off
  Display : Display
  Display1 : Display
  Energy 11 kV : MATLAB Function  TreatAsAtomicUnit=on
  HIF Logic Relay 11 KV : Subsystem  TreatAsAtomicUnit=on
  Integrator : Integrator
  Power 33 kV (Positive-Sequence)1 : spsPowerPositiveSequenceLib/Power (Positive-Sequence)  Freq=50  Vinit=[0, 0]  Iinit=[0, 0]  Ts=0
      link override Sequence Analyzer: Freq=50  seq=Negative
      link override Sequence Analyzer1: Freq=50  seq=Zero
      settings: SourceProductBaseCode=PS
  RMS1 : dspstat3/RMS  run=off  directionMode=Each column  dimension=1  InputProcessing=Columns as channels (frame based)  reset_popup=None
  RMS2 : dspstat3/RMS  run=off  directionMode=Each column  dimension=1  InputProcessing=Columns as channels (frame based)  reset_popup=None
  RMS3 : dspstat3/RMS  run=off  directionMode=Each column  dimension=1  InputProcessing=Columns as channels (frame based)  reset_popup=None
  Relational Operator1 : RelationalOperator  Operator=>  RndMeth=Nearest
  Scope{1..5,8,10} (7 alike) : Scope
  Scope12 : Scope  NumInputPorts=2
  Scope13 : Scope  NumInputPorts=3
  Scope15 : Scope  NumInputPorts=2
  C/S : Outport  VectorParamsAs1DForOutWhenUnconnected=off
  P11 kV : Outport  Port=2  VectorParamsAs1DForOutWhenUnconnected=off
  E 11kV : Outport  Port=3  VectorParamsAs1DForOutWhenUnconnected=off
  wires:
  Power 33 kV (Positive-Sequence)1/2 -> RMS3/1
  Iabc/1 -> Power 33 kV (Positive-Sequence)1/2
  RMS3/1 -> Scope5/1
  Energy 11 kV/1(Energy) -> RMS1/1
  Integrator/1 -> Scope3/1, Energy 11 kV/2(t)
  Power 33 kV (Positive-Sequence)1/1 -> RMS2/1
  Vabc/1 -> Power 33 kV (Positive-Sequence)1/1
  HIF Logic Relay 11 KV/1(Out1) -> C/S/1, Scope2/1
  Data Type Conversion1/1 -> Integrator/1
  Relational Operator1/1 -> Data Type Conversion1/1, Scope1/1
  Constant/1 -> Relational Operator1/2
  RMS2/1 -> Difference1/1, Scope13/1, Scope12/1, P11 kV/1, Scope4/1, Display/1
  Difference1/1 -> Scope13/2, Energy 11 kV/1(P), Scope15/1, Relational Operator1/1
  RMS1/1 -> Scope12/2, Scope15/2, Scope13/3, Display1/1, E 11kV/1, Scope10/1, Scope8/1, HIF Logic Relay 11 KV/3(In3), HIF Logic Relay 11 KV/2(In2), HIF Logic Relay 11 KV/1(In1)

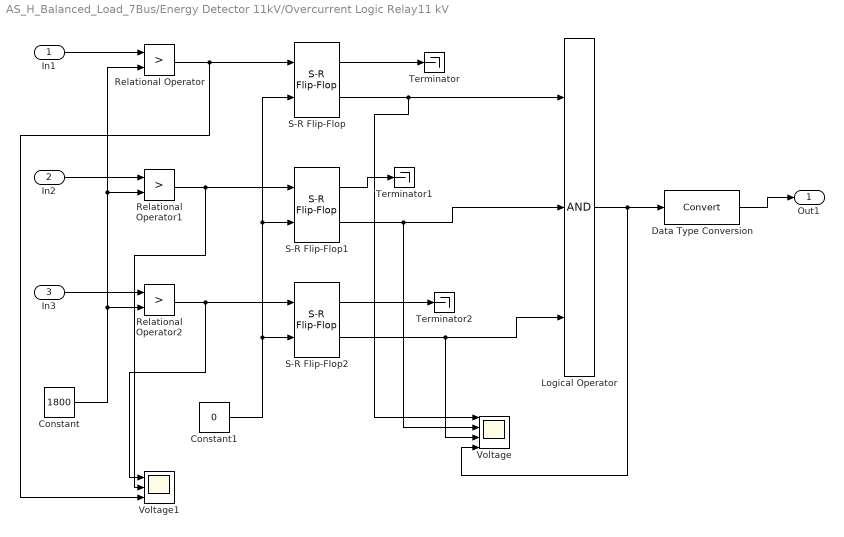
== system AS_H_Balanced_Load_7Bus/Energy Detector 11kV/Overcurrent Logic Relay11 kV  ==
  In1 : Inport
  In2 : Inport  Port=2
  In3 : Inport  Port=3
  Constant : Constant  Value=1800  VectorParams1D=off  OutDataTypeStr=Inherit: Inherit via back propagation  LockScale=on
  Constant1 : Constant  Value=0  VectorParams1D=off  OutDataTypeStr=Inherit: Inherit via back propagation  LockScale=on
  Data Type Conversion : DataTypeConversion
  Logical Operator : Logic  Inputs=3  AllPortsSameDT=off
  Relational Operator : RelationalOperator  Operator=>  RndMeth=Nearest
  Relational Operator1 : RelationalOperator  Operator=>  RndMeth=Nearest
  Relational Operator2 : RelationalOperator  Operator=>  RndMeth=Nearest
  S-R Flip-Flop : simulink_extras/Flip Flops/S-R Flip-Flop  initial_condition=0
  S-R Flip-Flop1 : simulink_extras/Flip Flops/S-R Flip-Flop  initial_condition=0
  S-R Flip-Flop2 : simulink_extras/Flip Flops/S-R Flip-Flop  initial_condition=0
  Terminator : Terminator
  Terminator1 : Terminator
  Terminator2 : Terminator
  Voltage : Scope  NumInputPorts=4
  Voltage1 : Scope  NumInputPorts=3
  Out1 : Outport  VectorParamsAs1DForOutWhenUnconnected=off
  wires:
  In1/1 -> Relational Operator/1
  In2/1 -> Relational Operator1/1
  In3/1 -> Relational Operator2/1
  Constant/1 -> Relational Operator2/2, Relational Operator1/2, Relational Operator/2
  Relational Operator/1 -> Voltage1/3, S-R Flip-Flop/1
  Relational Operator1/1 -> Voltage1/2, S-R Flip-Flop1/1
  Relational Operator2/1 -> Voltage1/1, S-R Flip-Flop2/1
  Constant1/1 -> S-R Flip-Flop2/2, S-R Flip-Flop1/2, S-R Flip-Flop/2
  S-R Flip-Flop/1 -> Terminator/1
  S-R Flip-Flop1/1 -> Terminator1/1
  S-R Flip-Flop2/1 -> Terminator2/1
  S-R Flip-Flop/2 -> Voltage/1, Logical Operator/1
  S-R Flip-Flop1/2 -> Voltage/2, Logical Operator/2
  S-R Flip-Flop2/2 -> Voltage/3, Logical Operator/3
  Data Type Conversion/1 -> Out1/1
  Logical Operator/1 -> Voltage/4, Data Type Conversion/1

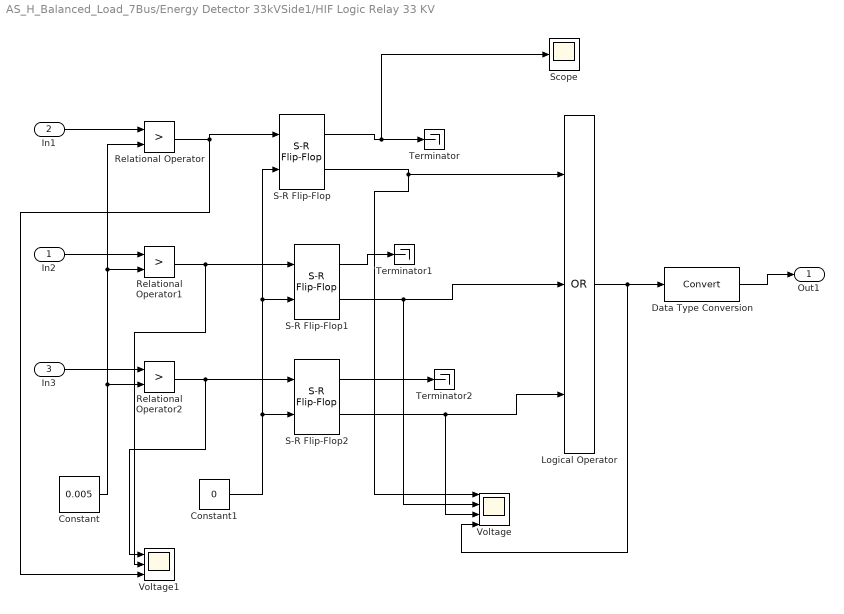
== system AS_H_Balanced_Load_7Bus/Energy Detector 33kVSide1/HIF Logic Relay 33 KV ==
  In2 : Inport
  In1 : Inport  Port=2
  In3 : Inport  Port=3
  Constant : Constant  Value=0.005  VectorParams1D=off  OutDataTypeStr=Inherit: Inherit via back propagation  LockScale=on
  Constant1 : Constant  Value=0  VectorParams1D=off  OutDataTypeStr=Inherit: Inherit via back propagation  LockScale=on
  Data Type Conversion : DataTypeConversion
  Logical Operator : Logic  Operator=OR  Inputs=3  AllPortsSameDT=off
  Relational Operator : RelationalOperator  Operator=>  RndMeth=Nearest
  Relational Operator1 : RelationalOperator  Operator=>  RndMeth=Nearest
  Relational Operator2 : RelationalOperator  Operator=>  RndMeth=Nearest
  S-R Flip-Flop : simulink_extras/Flip Flops/S-R Flip-Flop  initial_condition=0
  S-R Flip-Flop1 : simulink_extras/Flip Flops/S-R Flip-Flop  initial_condition=0
  S-R Flip-Flop2 : simulink_extras/Flip Flops/S-R Flip-Flop  initial_condition=0
  Scope : Scope
  Terminator : Terminator
  Terminator1 : Terminator
  Terminator2 : Terminator
  Voltage : Scope  NumInputPorts=4
  Voltage1 : Scope  NumInputPorts=3
  Out1 : Outport  VectorParamsAs1DForOutWhenUnconnected=off
  wires:
  In1/1 -> Relational Operator/1
  In2/1 -> Relational Operator1/1
  In3/1 -> Relational Operator2/1
  Constant/1 -> Relational Operator2/2, Relational Operator1/2, Relational Operator/2
  Relational Operator/1 -> Voltage1/3, S-R Flip-Flop/1
  Relational Operator1/1 -> Voltage1/2, S-R Flip-Flop1/1
  Relational Operator2/1 -> Voltage1/1, S-R Flip-Flop2/1
  Constant1/1 -> S-R Flip-Flop2/2, S-R Flip-Flop1/2, S-R Flip-Flop/2
  S-R Flip-Flop/1 -> Scope/1, Terminator/1
  S-R Flip-Flop1/1 -> Terminator1/1
  S-R Flip-Flop2/1 -> Terminator2/1
  S-R Flip-Flop/2 -> Voltage/1, Logical Operator/1
  S-R Flip-Flop1/2 -> Voltage/2, Logical Operator/2
  S-R Flip-Flop2/2 -> Voltage/3, Logical Operator/3
  Data Type Conversion/1 -> Out1/1
  Logical Operator/1 -> Voltage/4, Data Type Conversion/1

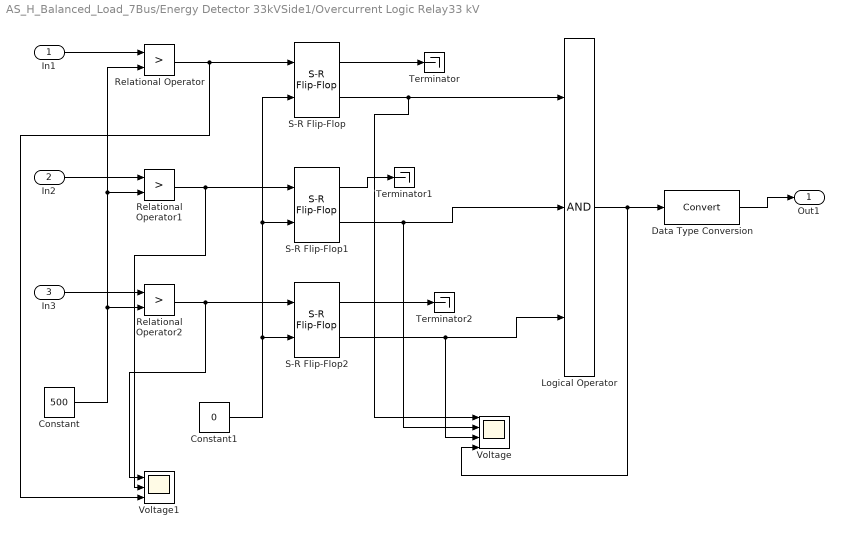
== system AS_H_Balanced_Load_7Bus/Energy Detector 33kVSide1/Overcurrent Logic Relay33 kV ==
  In1 : Inport
  In2 : Inport  Port=2
  In3 : Inport  Port=3
  Constant : Constant  Value=500  VectorParams1D=off  OutDataTypeStr=Inherit: Inherit via back propagation  LockScale=on
  Constant1 : Constant  Value=0  VectorParams1D=off  OutDataTypeStr=Inherit: Inherit via back propagation  LockScale=on
  Data Type Conversion : DataTypeConversion
  Logical Operator : Logic  Inputs=3  AllPortsSameDT=off
  Relational Operator : RelationalOperator  Operator=>  RndMeth=Nearest
  Relational Operator1 : RelationalOperator  Operator=>  RndMeth=Nearest
  Relational Operator2 : RelationalOperator  Operator=>  RndMeth=Nearest
  S-R Flip-Flop : simulink_extras/Flip Flops/S-R Flip-Flop  initial_condition=0
  S-R Flip-Flop1 : simulink_extras/Flip Flops/S-R Flip-Flop  initial_condition=0
  S-R Flip-Flop2 : simulink_extras/Flip Flops/S-R Flip-Flop  initial_condition=0
  Terminator : Terminator
  Terminator1 : Terminator
  Terminator2 : Terminator
  Voltage : Scope  NumInputPorts=4
  Voltage1 : Scope  NumInputPorts=3
  Out1 : Outport  VectorParamsAs1DForOutWhenUnconnected=off
  wires:
  In1/1 -> Relational Operator/1
  In2/1 -> Relational Operator1/1
  In3/1 -> Relational Operator2/1
  Constant/1 -> Relational Operator2/2, Relational Operator1/2, Relational Operator/2
  Relational Operator/1 -> Voltage1/3, S-R Flip-Flop/1
  Relational Operator1/1 -> Voltage1/2, S-R Flip-Flop1/1
  Relational Operator2/1 -> Voltage1/1, S-R Flip-Flop2/1
  Constant1/1 -> S-R Flip-Flop2/2, S-R Flip-Flop1/2, S-R Flip-Flop/2
  S-R Flip-Flop/1 -> Terminator/1
  S-R Flip-Flop1/1 -> Terminator1/1
  S-R Flip-Flop2/1 -> Terminator2/1
  S-R Flip-Flop/2 -> Voltage/1, Logical Operator/1
  S-R Flip-Flop1/2 -> Voltage/2, Logical Operator/2
  S-R Flip-Flop2/2 -> Voltage/3, Logical Operator/3
  Data Type Conversion/1 -> Out1/1
  Logical Operator/1 -> Voltage/4, Data Type Conversion/1

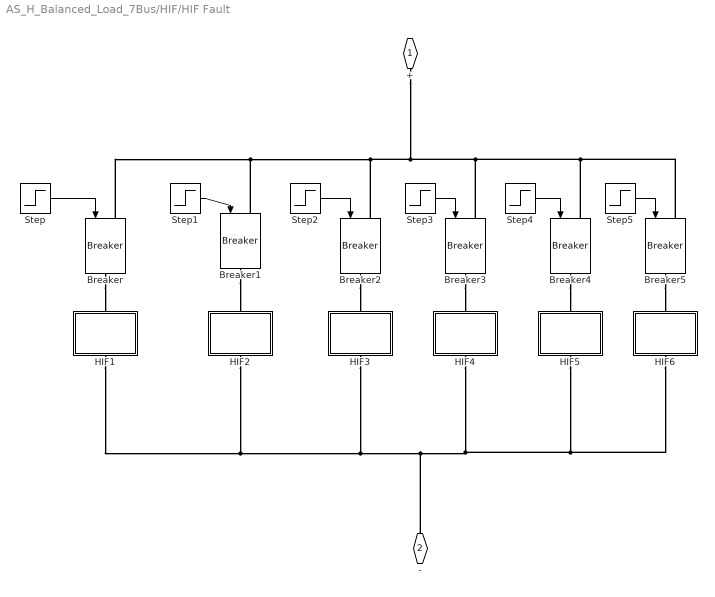
== system AS_H_Balanced_Load_7Bus/HIF/HIF Fault ==
  Breaker{,1..5} (6 alike) : spsBreakerLib/Breaker  InitialState=0  SwitchingTimes="[1/50  5/50]"  External=on  BreakerResistance=0.01  SnubberResistance=1e6  SnubberCapacitance=inf  Measurements=Branch voltage and current  MoreParameters=on  NoBreakLoop=off
      settings: SourceProductBaseCode=PS
  HIF1 : Subsystem
  HIF2 : Subsystem
  HIF3 : Subsystem
  HIF4 : Subsystem
  HIF5 : Subsystem
  HIF6 : Subsystem
  Step : Step  Time=0.01  SampleTime=0.001  ZeroCross=off
  Step1 : Step  Time=0.12  SampleTime=0.001  ZeroCross=off
  Step2 : Step  Time=0.14  SampleTime=0.001  ZeroCross=off
  Step3 : Step  Time=0.16  SampleTime=0.001  ZeroCross=off
  Step4 : Step  Time=0.18  SampleTime=0.001  VectorParams1D=off
  Step5 : Step  Time=0.2  SampleTime=0.001  VectorParams1D=off
  + : PMIOPort  Side=Left
  - : PMIOPort  Port=2  Side=Right
  wires:
  Step4/1 -> Breaker4/1
  Step1/1 -> Breaker1/1
  Step2/1 -> Breaker2/1
  Step3/1 -> Breaker3/1
  Step/1 -> Breaker/1
  Step5/1 -> Breaker5/1
  connections:
  Breaker/LConn1 -- Breaker1/LConn1 -- Breaker2/LConn1 -- Breaker5/LConn1 -- Breaker4/LConn1 -- Breaker3/LConn1 -- +/RConn1
  Breaker/RConn1 -- HIF1/LConn1
  Breaker4/RConn1 -- HIF5/LConn1
  Breaker5/RConn1 -- HIF6/LConn1
  Breaker3/RConn1 -- HIF4/LConn1
  Breaker2/RConn1 -- HIF3/LConn1
  HIF5/RConn1 -- HIF6/RConn1 -- HIF4/RConn1 -- HIF3/RConn1 -- HIF2/RConn1 -- HIF1/RConn1 -- -/RConn1
  Breaker1/RConn1 -- HIF2/LConn1

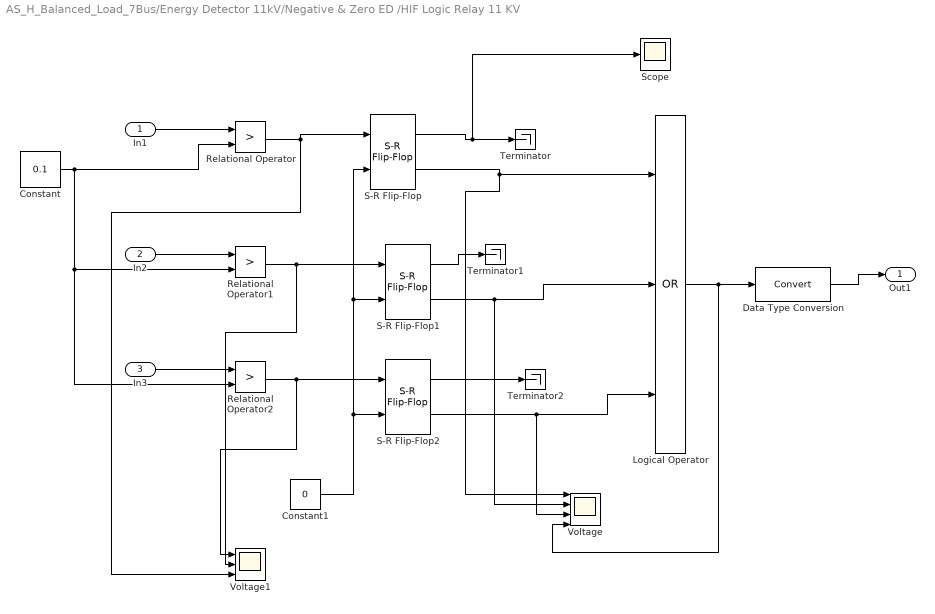
== system AS_H_Balanced_Load_7Bus/Energy Detector 11kV/Negative & Zero ED /HIF Logic Relay 11 KV ==
  In1 : Inport
  In2 : Inport  Port=2
  In3 : Inport  Port=3
  Constant : Constant  Value=0.1  VectorParams1D=off  OutDataTypeStr=Inherit: Inherit via back propagation  LockScale=on
  Constant1 : Constant  Value=0  VectorParams1D=off  OutDataTypeStr=Inherit: Inherit via back propagation  LockScale=on
  Data Type Conversion : DataTypeConversion
  Logical Operator : Logic  Operator=OR  Inputs=3  AllPortsSameDT=off
  Relational Operator : RelationalOperator  Operator=>  RndMeth=Nearest
  Relational Operator1 : RelationalOperator  Operator=>  RndMeth=Nearest
  Relational Operator2 : RelationalOperator  Operator=>  RndMeth=Nearest
  S-R Flip-Flop : simulink_extras/Flip Flops/S-R Flip-Flop  initial_condition=0
  S-R Flip-Flop1 : simulink_extras/Flip Flops/S-R Flip-Flop  initial_condition=0
  S-R Flip-Flop2 : simulink_extras/Flip Flops/S-R Flip-Flop  initial_condition=0
  Scope : Scope
  Terminator : Terminator
  Terminator1 : Terminator
  Terminator2 : Terminator
  Voltage : Scope  NumInputPorts=4
  Voltage1 : Scope  NumInputPorts=3
  Out1 : Outport  VectorParamsAs1DForOutWhenUnconnected=off
  wires:
  In1/1 -> Relational Operator/1
  In2/1 -> Relational Operator1/1
  In3/1 -> Relational Operator2/1
  Constant/1 -> Relational Operator2/2, Relational Operator1/2, Relational Operator/2
  Relational Operator/1 -> Voltage1/3, S-R Flip-Flop/1
  Relational Operator1/1 -> Voltage1/2, S-R Flip-Flop1/1
  Relational Operator2/1 -> Voltage1/1, S-R Flip-Flop2/1
  Constant1/1 -> S-R Flip-Flop2/2, S-R Flip-Flop1/2, S-R Flip-Flop/2
  S-R Flip-Flop/1 -> Scope/1, Terminator/1
  S-R Flip-Flop1/1 -> Terminator1/1
  S-R Flip-Flop2/1 -> Terminator2/1
  S-R Flip-Flop/2 -> Voltage/1, Logical Operator/1
  S-R Flip-Flop1/2 -> Voltage/2, Logical Operator/2
  S-R Flip-Flop2/2 -> Voltage/3, Logical Operator/3
  Data Type Conversion/1 -> Out1/1
  Logical Operator/1 -> Voltage/4, Data Type Conversion/1

== system AS_H_Balanced_Load_7Bus/HIF/HIF Fault/HIF1 ==
  DC Voltage Source : spsDCVoltageSourceLib/DC Voltage Source  Amplitude=1800  Measurements=None
  DC Voltage Source1 : spsDCVoltageSourceLib/DC Voltage Source  Amplitude=2700  Measurements=None
  Diode : spsDiodeLib/Diode  Ron=0.001  Lon=0  Vf=0.8  IC=0  UseSnubber=off  Rs=500  Cs=250e-9  Measurements=on
  Diode1 : spsDiodeLib/Diode  Ron=0.001  Lon=0  Vf=0.8  IC=0  UseSnubber=off  Rs=500  Cs=250e-9  Measurements=on
  Series RLC Branch : spsSeriesRLCBranchLib/Series RLC Branch  LConnTagsString=__new0  RConnTagsString=__new0  BranchType=R  Resistance=500  Inductance=1e-3  SetiL0=off  InitialCurrent=0  Capacitance=1e-6  Setx0=off  InitialVoltage=0  Measurements=None
  Series RLC Branch1 : spsSeriesRLCBranchLib/Series RLC Branch  LConnTagsString=__new0  RConnTagsString=__new0  BranchType=R  Resistance=500  Inductance=1e-3  SetiL0=off  InitialCurrent=0  Capacitance=1e-6  Setx0=off  InitialVoltage=0  Measurements=None
  Terminator : Terminator
  Terminator1 : Terminator
  + : PMIOPort  Side=Left
  - : PMIOPort  Port=2  Side=Right
  wires:
  Diode/1 -> Terminator/1
  Diode1/1 -> Terminator1/1
  connections:
  Series RLC Branch1/RConn1 -- Diode/LConn1
  DC Voltage Source1/RConn1 -- Diode/RConn1
  DC Voltage Source/RConn1 -- DC Voltage Source1/LConn1 -- -/RConn1
  Series RLC Branch/RConn1 -- Diode1/RConn1
  Series RLC Branch1/LConn1 -- +/RConn1 -- Series RLC Branch/LConn1
  DC Voltage Source/LConn1 -- Diode1/LConn1

== system AS_H_Balanced_Load_7Bus/HIF/HIF Fault/HIF2 ==
  DC Voltage Source : spsDCVoltageSourceLib/DC Voltage Source  Amplitude=1800  Measurements=None
  DC Voltage Source1 : spsDCVoltageSourceLib/DC Voltage Source  Amplitude=2800  Measurements=None
  Diode : spsDiodeLib/Diode  Ron=0.001  Lon=0  Vf=0.8  IC=0  UseSnubber=off  Rs=500  Cs=250e-9  Measurements=on
  Diode1 : spsDiodeLib/Diode  Ron=0.001  Lon=0  Vf=0.8  IC=0  UseSnubber=off  Rs=500  Cs=250e-9  Measurements=on
  Series RLC Branch : spsSeriesRLCBranchLib/Series RLC Branch  LConnTagsString=__new0  RConnTagsString=__new0  BranchType=R  Resistance=520  Inductance=1e-3  SetiL0=off  InitialCurrent=0  Capacitance=1e-6  Setx0=off  InitialVoltage=0  Measurements=None
  Series RLC Branch1 : spsSeriesRLCBranchLib/Series RLC Branch  LConnTagsString=__new0  RConnTagsString=__new0  BranchType=R  Resistance=520  Inductance=1e-3  SetiL0=off  InitialCurrent=0  Capacitance=1e-6  Setx0=off  InitialVoltage=0  Measurements=None
  Terminator : Terminator
  Terminator1 : Terminator
  + : PMIOPort  Side=Left
  - : PMIOPort  Port=2  Side=Right
  wires:
  Diode/1 -> Terminator/1
  Diode1/1 -> Terminator1/1
  connections:
  Series RLC Branch1/RConn1 -- Diode/LConn1
  DC Voltage Source1/RConn1 -- Diode/RConn1
  DC Voltage Source1/LConn1 -- DC Voltage Source/RConn1 -- -/RConn1
  Series RLC Branch/RConn1 -- Diode1/RConn1
  Series RLC Branch/LConn1 -- Series RLC Branch1/LConn1 -- +/RConn1
  DC Voltage Source/LConn1 -- Diode1/LConn1

== system AS_H_Balanced_Load_7Bus/HIF/HIF Fault/HIF3 ==
  DC Voltage Source : spsDCVoltageSourceLib/DC Voltage Source  Amplitude=1900  Measurements=None
  DC Voltage Source1 : spsDCVoltageSourceLib/DC Voltage Source  Amplitude=2900  Measurements=None
  Diode : spsDiodeLib/Diode  Ron=0.001  Lon=0  Vf=0.8  IC=0  UseSnubber=off  Rs=500  Cs=250e-9  Measurements=on
  Diode1 : spsDiodeLib/Diode  Ron=0.001  Lon=0  Vf=0.8  IC=0  UseSnubber=off  Rs=500  Cs=250e-9  Measurements=on
  Series RLC Branch : spsSeriesRLCBranchLib/Series RLC Branch  LConnTagsString=__new0  RConnTagsString=__new0  BranchType=R  Resistance=540  Inductance=1e-3  SetiL0=off  InitialCurrent=0  Capacitance=1e-6  Setx0=off  InitialVoltage=0  Measurements=None
  Series RLC Branch1 : spsSeriesRLCBranchLib/Series RLC Branch  LConnTagsString=__new0  RConnTagsString=__new0  BranchType=R  Resistance=540  Inductance=1e-3  SetiL0=off  InitialCurrent=0  Capacitance=1e-6  Setx0=off  InitialVoltage=0  Measurements=None
  Terminator : Terminator
  Terminator1 : Terminator
  + : PMIOPort  Side=Left
  - : PMIOPort  Port=2  Side=Right
  wires:
  Diode/1 -> Terminator/1
  Diode1/1 -> Terminator1/1
  connections:
  Series RLC Branch1/RConn1 -- Diode/LConn1
  DC Voltage Source1/RConn1 -- Diode/RConn1
  DC Voltage Source1/LConn1 -- DC Voltage Source/RConn1 -- -/RConn1
  Series RLC Branch/RConn1 -- Diode1/RConn1
  Series RLC Branch/LConn1 -- Series RLC Branch1/LConn1 -- +/RConn1
  DC Voltage Source/LConn1 -- Diode1/LConn1
